simulink model "HapticMasterVR_mojakopija"  (R2019b)
settings: Solver=FixedStepDiscrete  StartTime=0.0  StopTime=20  RelTol=1e-3  EnableMultiTasking=on
undefined symbols (not defined in the file or in its folder): DiscIntNeverNeededParam, dT, fbGain, q0
libraries: simulink x1, vrlib x1
Description:
  | Real-Time Van der Pol Simulation
  | 
  | This demonstration shows a real-time version of the Simulink Van der Pol
  | simulation demo. This model does not need any external signals, so it does
  | not need any data acquisition hardware or driver. This makes the model ideal
  | for first experiments with Real-Time Windows Target, without need to
  | worry about proper I/O hardware configuration.
  | 
  | How to run this demo:
  | 
  |   1. Build the model using Tools -> Real-Time Workshop -> Build Model.
  |   2. Connect to the real-time code using Simulation -> Connect to target.
  |   3. Start the real-time execution using Simulation -> Start real-time code.
settings Model: EnablePacing=on  Creator=Houska  LastModifiedBy=student
settings DataIOCC: LimitDataPoints=on  SaveFormat=Array  SignalLoggingSaveFormat=ModelDataLogs  SaveOutput=off  SaveTime=off  ReturnWorkspaceOutputs=off  SignalLoggingName=logsOut
settings OptimizationCC: ExpressionDepthLimit=2147483647  InitFltsAndDblsToZero=on  LifeSpan=inf
settings DebuggingCC: SaveWithParameterizedLinksMsg=none  UnderspecifiedInitializationDetection=Classic  MergeDetectMultiDrivingBlocksExec=none  SignalResolutionControl=TryResolveAllWithWarning  MultiTaskDSMMsg=warning  MultiTaskCondExecSysMsg=none  FcnCallInpInsideContextMsg=warning  StateNameClashWarn=warning  SFUnexpectedBacktrackingDiag=warning  SFNoUnconditionalDefaultTransitionDiag=warning  SFExecutionAtInitializationDiag=none  ArithmeticOperatorsInVariantConditions=warning
settings HardwareCC: ProdBitPerPointer=32  ProdBitPerSizeT=32  ProdBitPerPtrDiffT=32  ProdLargestAtomicFloat=None  ProdWordSize=32  ProdHWDeviceType=32-bit Real-Time Windows Target
settings ModelReferenceCC: PropagateSignalLabelsOutOfModel=off
settings SFSimCC: SimUseLocalCustomCode=off  CustomCodeUndefinedFunction=UseInterfaceOnly
settings RTWCC: Description=Real-Time Windows Target  SystemTargetFile=rtwin.tlc  TemplateMakefile=rtwin.tmf  RTWUseLocalCustomCode=off
settings CodeAppCC: StateflowObjectComments=on
settings TargetCC: TargetFcnLib=ansi_tfl_tmw.mat  ModelReferenceCompliant=off  CompOptLevelCompliant=off  PreserveStateflowLocalDataDimensions=off
settings ConfigComp: CovMetricSettings=dw  CovHtmlReporting=on  CovSaveCumulativeToWorkspaceVar=on  CovSaveSingleToWorkspaceVar=on  CovExternalEMLEnable=off  CovSFcnEnable=off

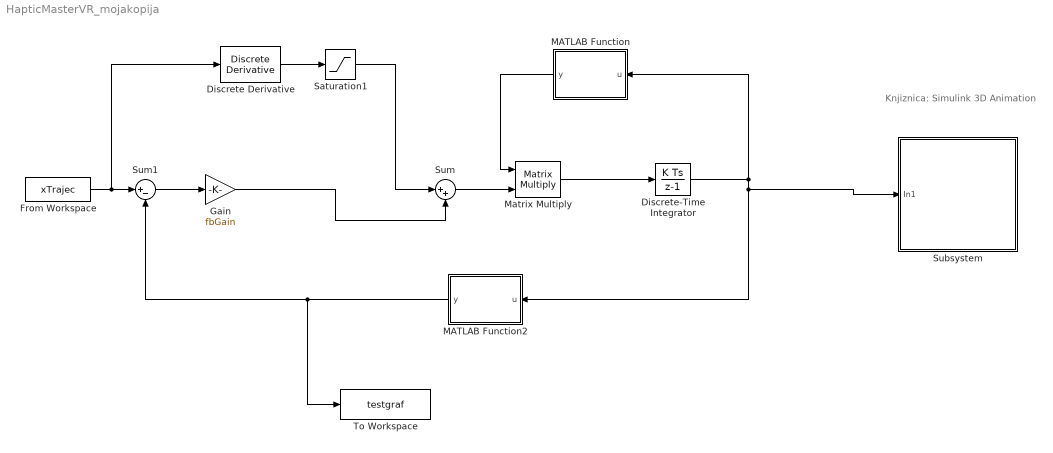
== system HapticMasterVR_mojakopija ==
  note: Knjiznica: Simulink 3D Animation
  Discrete Derivative : simulink/Discrete/Discrete Derivative  gainval=1.0  ICPrevScaledInput=0.0  OutMin=[]  OutMax=[]  OutDataType=fixdt(1, 16)  OutScaling=2^-10  DoSatur=off
  Discrete-Time Integrator : DiscreteIntegrator  InitialCondition=q0  SampleTime=dT  ICPrevOutput=DiscIntNeverNeededParam  ICPrevScaledInput=DiscIntNeverNeededParam
  From Workspace : FromWorkspace  VariableName=xTrajec  SampleTime=0
  Gain : Gain  Gain=fbGain
  MATLAB Function : MATLAB Function  TreatAsAtomicUnit=on
  MATLAB Function2 : MATLAB Function  TreatAsAtomicUnit=on
  Matrix Multiply : Product  Multiplication=Matrix(*)
  Saturation1 : Saturate
  Subsystem : Subsystem
      mask Display:
      | image(imread('HapticMaster.png'))
      | color('white')
      | port_label('input',1, 'q')
  Sum : Sum  Inputs=|++
  Sum1 : Sum  Inputs=|+-
  To Workspace : ToWorkspace  VariableName=testgraf  SampleTime=-1
  wires:
  MATLAB Function/1(y) -> Matrix Multiply/1
  Gain/1 -> Sum/2
  Matrix Multiply/1 -> Discrete-Time Integrator/1
  Sum/1 -> Matrix Multiply/2
  Saturation1/1 -> Sum/1
  Discrete Derivative/1 -> Saturation1/1
  From Workspace/1 -> Discrete Derivative/1, Sum1/1
  Sum1/1 -> Gain/1
  Discrete-Time Integrator/1 -> Subsystem/1(In1), MATLAB Function2/1(u), MATLAB Function/1(u)
  MATLAB Function2/1(y) -> To Workspace/1, Sum1/2

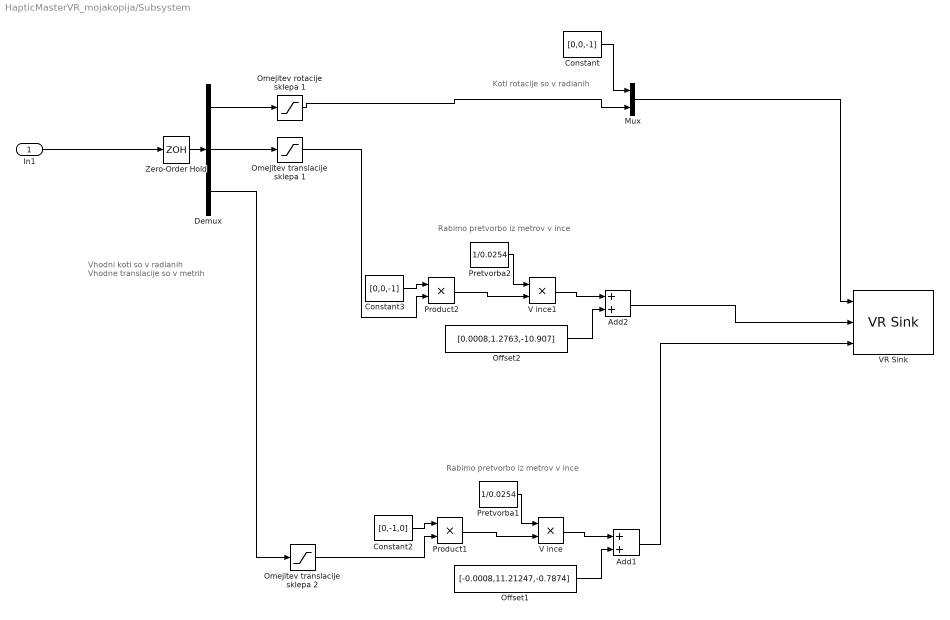
== system HapticMasterVR_mojakopija/Subsystem ==
  note: Koti rotacije so v radianih
  note: Vhodni koti so v radianih
      | Vhodne translacije so v metrih
  note: Rabimo pretvorbo iz metrov v ince
  note: Rabimo pretvorbo iz metrov v ince
  In1 : Inport
  Add1 : Sum
  Add2 : Sum
  Constant : Constant  Value=[0,0,-1]  SampleTime=-1
  Constant2 : Constant  Value=[0,-1,0]  SampleTime=-1
  Constant3 : Constant  Value=[0,0,-1]  SampleTime=-1
  Demux : Demux  Outputs=3
  Mux : Mux  Inputs=2
  Offset1 : Constant  Value=[-0.0008,11.21247,-0.7874]  SampleTime=-1
  Offset2 : Constant  Value=[0.0008,1.2763,-10.907]  SampleTime=-1
  Omejitev rotacije sklepa 1 : Saturate  UpperLimit=30  LowerLimit=-30
  Omejitev translacije sklepa 1 : Saturate  UpperLimit=0.45729/2  LowerLimit=-0.45729/2
  Omejitev translacije sklepa 2 : Saturate  UpperLimit=0.3797/2  LowerLimit=-0.3797/2
  Pretvorba1 : Constant  Value=1/0.0254  SampleTime=-1
  Pretvorba2 : Constant  Value=1/0.0254  SampleTime=-1
  Product1 : Product  RndMeth=Zero
  Product2 : Product  RndMeth=Zero
  V ince : Product  RndMeth=Zero
  V ince1 : Product  RndMeth=Zero
  VR Sink : vrlib/VR Sink  InstantiateOnLoad=on  SampleTime=0.05  ViewEnable=on  RemoteChange=off  RemoteView=on  FieldsWritten=HM_01.rotation.4.1.1.double#HM_01.translation.3.1.1.double#HM_02.translation.3.1.1.double  WorldFileName=HapticMaster.wrl  AutoView=on  VideoDimensions=[]  AllowVariableSize=off  FigureProperties="{'Position', 'Name', 'Viewpoint', 'CameraBound', 'CameraDirection', 'CameraPosition', 'CameraUpVector', 'ZoomFactor', 'Antialiasing', 'Headlight', 'Lighting', 'NavPanel', 'Sound', 'StatusBar', 'Stereo3D', 'Stereo3DCameraOffset', 'Stereo3DHIT', 'ToolBar', 'Textures', 'Transparency', 'Triad', 'Wireframe', 'NavZones', 'NavMode', 'NavSpeed', 'CaptureFileFormat', 'CaptureFileName', 'Record2DCompressMethod', 'Record2DCompressQuality', 'Record2D', 'Record2DFileName', 'Record2DFPS'; [1.7000000000000000e+01   8.8000000000000000e+01   5.7600000000000000e+02   3.5000000000000000e+02], '', '_untitled_1', 'on', [2.0816681711721685e-17   0.0000000000000000e+00  -1.0000000000000004e+00], [0.0000000000000000e+00   0.0000000000000000e+00  -4.0000000000000000e+00], [0.0000000000000000e+00   1.0000000000000000e+00   0.0000000000000000e+00], [1.0000000000000000e+00], 'on', 'on', 'on', 'halfbar', 'on', 'on', 'off', [1.0000000149011612e-01], [0.0000000000000000e+00], 'on', 'on', 'on', 'none', 'off', 'off', 'fly', 'normal', 'tif', '%f_anim_%n.tif', 'auto', [7.5000000000000000e+01], 'off', '%f_anim_%n.avi', 'auto'}"
      settings: SourceProductName=Simulink
  Zero-Order Hold : ZeroOrderHold  SampleTime=0.05
  wires:
  Constant/1 -> Mux/1
  In1/1 -> Zero-Order Hold/1
  Zero-Order Hold/1 -> Demux/1
  Constant2/1 -> Product1/1
  Offset1/1 -> Add1/2
  Add1/1 -> VR Sink/3
  Demux/1 -> Omejitev rotacije sklepa 1/1
  Mux/1 -> VR Sink/1
  Product1/1 -> V ince/2
  V ince/1 -> Add1/1
  Pretvorba1/1 -> V ince/1
  Constant3/1 -> Product2/1
  Offset2/1 -> Add2/2
  Product2/1 -> V ince1/2
  V ince1/1 -> Add2/1
  Pretvorba2/1 -> V ince1/1
  Add2/1 -> VR Sink/2
  Demux/2 -> Omejitev translacije sklepa 1/1
  Omejitev rotacije sklepa 1/1 -> Mux/2
  Demux/3 -> Omejitev translacije sklepa 2/1
  Omejitev translacije sklepa 1/1 -> Product2/2
  Omejitev translacije sklepa 2/1 -> Product1/2

== matlab function HapticMasterVR_mojakopija/MATLAB Function ==
  data: u input; y output
function y = invJa(u)

y = ijacZYZeul(u);

== matlab function HapticMasterVR_mojakopija/MATLAB Function2 ==
  data: u input; y output
function y = dirkin(u)

y1 = q2ZYZeul(u);
y = y1(1:3)
